simulink model "pulsestep"  (Simulink 2.09)
settings: Solver=ode45  StartTime=0.0  StopTime=0.5  RelTol=1e-3  AbsTol=1e-6
libraries: simulink x1
settings Model: ConsistencyChecking=off  RTWTemplateMakefile=grt_vc.tmf

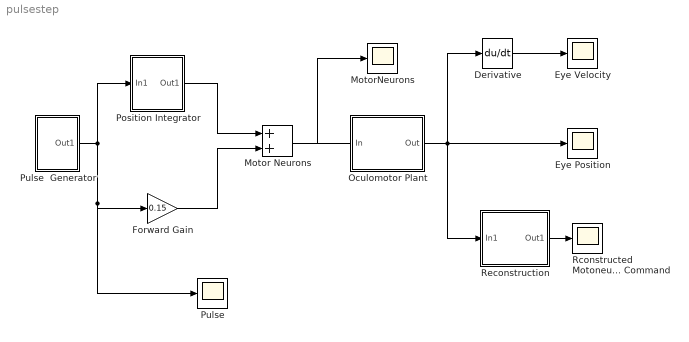
== system pulsestep ==
  Derivative : Derivative
  Eye Position : Scope
      settings: TickLabels=on  TimeRange=auto  YMin=-10  YMax=50  SaveToWorkspace=off  SaveName=ScopeData
  Eye Velocity : Scope
      settings: TickLabels=on  TimeRange=auto  YMin=-100  YMax=800  SaveToWorkspace=off  SaveName=ScopeData
  Forward Gain : Gain  Gain=0.15
  Motor Neurons : Sum  Inputs=++
  MotorNeurons : Scope
      settings: TickLabels=on  TimeRange=auto  YMin=-10  YMax=150  SaveToWorkspace=off  SaveName=ScopeData
  Oculomotor Plant : Subsystem  mask(Oculomotor Plant){T1=0.15, T2=0.012}
      mask prompts: T1 "High Time Constant (T1)"; T2 "Low Time Constant (T2)"
      mask help:
      | Second order model of the oculomotor plant
      | as proposed by Robinson and colleagues.
      |
      |  Model equation in Laplace notation:
      |
      |                         1
      |  H(s) = ---------------
      |             (1 + s.T1) . (1 + s.T2)
      mask Help:
      | T1 is the `high' time constant (muscle twitch relaxation time)
      |       default value: 0.15 sec
      |  T2 is the `low' time constant (muscle twitch contraction time)
      |       default value: 0.012 sec
      mask Display:
      | plot([0 0.1 0.15 0.2 0.25 0.3 0.5 0.7 0.9 1], [0 0.1 0.4 0.65 0.66 0.55 0.35 0.15 0.05 0])
      | text(0.04,0.5,'T2') text(0.55,0.5, 'T1')
  Position Integrator : Subsystem  mask(Eye Position Integrator){G=1}
      mask prompts: G "Integrator Gain"
      mask Display: text(.35,.5,'INT')
  Pulse : Scope
      settings: TickLabels=on  TimeRange=auto  YMin=-100  YMax=800  SaveToWorkspace=off  SaveName=ScopeData
  Pulse  Generator : Subsystem  mask(Pulse){D=60, P=600}
      mask prompts: D "Pulse Duration [ms]"; P "Pulse Height [200-800]"
      mask Display: plot([0.05 0.3 0.305 0.6 0.605 0.9],[0.1 0.1 0.7 0.7 0.1 0.1])
  Rconstructed Motoneuron Command : Scope
      settings: TickLabels=on  TimeRange=auto  YMin=-10  YMax=150  SaveToWorkspace=off  SaveName=ScopeData
  Reconstruction : Subsystem  mask(Inverse Plant Model){T2=0.012, T1=0.15}
      mask prompts: T2 "Short Time Constant (s)"; T1 "Long Time Constant (s)"
      mask help:
      | Inverse model of the plant, that reconstructs the pulse-step motoneuron command from an eye position input signal.
      | You may enter the long and short time constants.
      | Typically, these would be the same as the original plant parameters.
      |
      | However, you may wish to study the effect of the time constants on the reconstruction of motoneuron activity, by choosing slightly different values.
      mask Display:
      | text(0.2,0.8,'INVERSE')
      | text(0.3,0.6,'PLANT')
      | text(0.25,0.4,'MODEL')
  wires:
  Reconstruction/1(Out1) -> Rconstructed Motoneuron Command/1
  Derivative/1 -> Eye Velocity/1
  Oculomotor Plant/1(Out) -> Reconstruction/1(In1), Derivative/1, Eye Position/1
  Position Integrator/1(Out1) -> Motor Neurons/1
  Forward Gain/1 -> Motor Neurons/2
  Motor Neurons/1 -> MotorNeurons/1, Oculomotor Plant/1("In ")
  Pulse  Generator/1(Out1) -> Position Integrator/1(In1), Pulse/1, Forward Gain/1

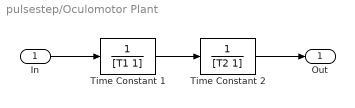
== system pulsestep/Oculomotor Plant ==
  "In " : Inport  Port=1  PortWidth=-1  SampleTime=-1
  Time Constant 1 : TransferFcn  Numerator=[1]  Denominator=[T1 1]
  Time Constant 2 : TransferFcn  Numerator=[1]  Denominator=[T2 1]
  Out : Outport  Port=1  InitialOutput=0
  wires:
  Time Constant 2/1 -> Out/1
  "In "/1 -> Time Constant 1/1
  Time Constant 1/1 -> Time Constant 2/1

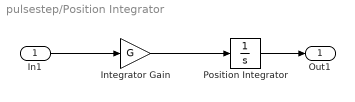
== system pulsestep/Position Integrator ==
  In1 : Inport  Port=1  PortWidth=-1  SampleTime=-1
  Integrator Gain : Gain  Gain=G
  Position Integrator : Integrator  ExternalReset=none  InitialConditionSource=internal  InitialCondition=0  LimitOutput=off  UpperSaturationLimit=inf  LowerSaturationLimit=-inf  ShowSaturationPort=off  ShowStatePort=off  AbsoluteTolerance=auto
  Out1 : Outport  Port=1  InitialOutput=0
  wires:
  Integrator Gain/1 -> Position Integrator/1
  Position Integrator/1 -> Out1/1
  In1/1 -> Integrator Gain/1

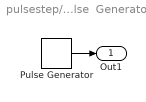
== system pulsestep/Pulse  Generator ==
  Pulse Generator : simulink/Sources/Pulse Generator  period=1  duty=D / 10  amplitude=P  start=0.1
  Out1 : Outport  Port=1  InitialOutput=0
  wires:
  Pulse Generator/1 -> Out1/1

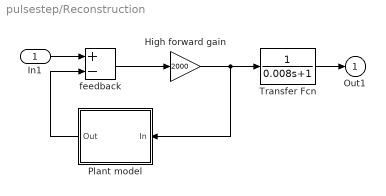
== system pulsestep/Reconstruction ==
  In1 : Inport  Port=1  PortWidth=-1  SampleTime=-1
  High forward gain : Gain  Gain=2000
  Plant model : Subsystem  Orientation=left  mask(Oculomotor Plant){T1=T1, T2=T2}
      mask prompts: T1 "High Time Constant (T1)"; T2 "Low Time Constant (T2)"
      mask help:
      | Second order model of the oculomotor plant
      | as proposed by Robinson and colleagues.
      |
      |  Model equation in Laplace notation:
      |
      |                         1
      |  H(s) = ---------------
      |             (1 + s.T1) . (1 + s.T2)
      mask Help:
      | T1 is the `high' time constant (muscle twitch relaxation time)
      |       default value: 0.15 sec
      |  T2 is the `low' time constant (muscle twitch contraction time)
      |       default value: 0.012 sec
      mask Display:
      | plot([0 0.1 0.15 0.2 0.25 0.3 0.5 0.7 0.9 1], [0 0.1 0.4 0.65 0.66 0.55 0.35 0.15 0.05 0])
      | text(0.04,0.5,'T2') text(0.55,0.5, 'T1')
  Transfer Fcn : TransferFcn  Numerator=[1]  Denominator=[0.008 1]
  feedback : Sum  Inputs=+-
  Out1 : Outport  Port=1  InitialOutput=0
  wires:
  High forward gain/1 -> Plant model/1("In "), Transfer Fcn/1
  Transfer Fcn/1 -> Out1/1
  In1/1 -> feedback/1
  Plant model/1(Out) -> feedback/2
  feedback/1 -> High forward gain/1

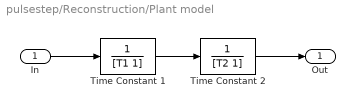
== system pulsestep/Reconstruction/Plant model ==
  "In " : Inport  Port=1  PortWidth=-1  SampleTime=-1
  Time Constant 1 : TransferFcn  Numerator=[1]  Denominator=[T1 1]
  Time Constant 2 : TransferFcn  Numerator=[1]  Denominator=[T2 1]
  Out : Outport  Port=1  InitialOutput=0
  wires:
  Time Constant 2/1 -> Out/1
  "In "/1 -> Time Constant 1/1
  Time Constant 1/1 -> Time Constant 2/1
